simulink model "regulator"  (R2023a)
settings: Solver=VariableStepAuto  StartTime=0.0  StopTime=1250  RelTol=1e-3
values from neighbouring files (symbols this model uses):
  A = [   a11,    0,      0,      0 ... (first row only)    [linearize_4tanks.m]    (also in parameters.mat = [-0.0171366511824 0.0171366511824 0 0 0 -0.0952465397017 0 0)
  A_kf = [-0.0171366511824 0.0171366511824 0 0 -0.405989384527 -1.0114279511 -4.63493813994e-17 -1.85727570483e-16 0 0 -0.052376732387 0.052376732387 ... (16 elements, 4x4)]    [parameters.mat]
  B = [   0,      b12 ... (first row only)    [linearize_4tanks.m]    (also in parameters.mat = [0  0.0970102697521; 0.120715699163  0; 0.138722651778  0; 0)
  B_kf = [0 0.120715699163 0.138722651778 0 0.0970102697521 0 0 0.159450121706 0.405989384527 0.916181411394 4.63493813994e-17 1.85727570483e-16 ... (16 elements, 4x4)]    [parameters.mat]
  C = [   0,      1,      0,      0 ... (first row only)    [linearize_4tanks.m]    (also in parameters.mat = [0  1  0  0; 0  0  0  1])
  C_kf = [1 0 0 0 0 1 0 0 0 0 1 0 ... (16 elements, 4x4)]    [parameters.mat]
  D_kf = [0 0 0 0 0 0 0 0 0 0 0 0 ... (16 elements, 4x4)]    [parameters.mat]
  K_integrators = [-0.0995479981451  -0.00949716090787; 0.00949716090787  -0.0995479981451]    [parameters.mat]
  K_state = [0.12950650673  0.722856465098  0.0139705767535  0.0637209208421; -0.0211766819284  -0.0833619871599  0.236348353203  0.657206774714]    [parameters.mat]
  u_bar = reshape(z_opt(5:6), [2, 1])    [linearize_4tanks.m]    (also in parameters.mat = [6.60003195923 9.28189672086])
  x_bar = reshape(z_opt(1:4), [4, 1])    [linearize_4tanks.m]    (also in parameters.mat = [24.6597369405 10 3.03378366821 10])
undefined symbols (not defined in the file or in its folder): DiscIntNeverNeededParam
libraries: discretizing x2
settings Model: Creator=ermarinellone  LastModifiedBy=ermarinellone

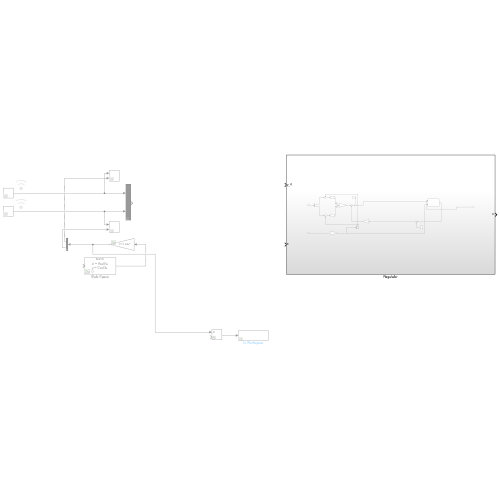
[thumbnail: Simulink's stored preview of the top-level diagram]
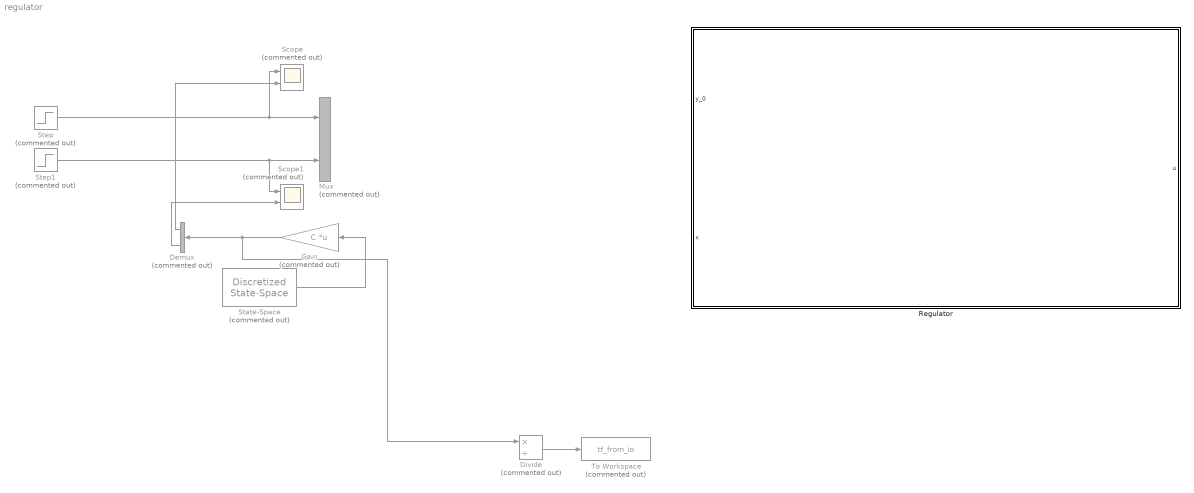
== system regulator ==
  Demux : Demux  Commented=on  Outputs=2
  Divide : Product  Commented=on  Inputs=*/
  Gain : Gain  Commented=on  Gain=C  Multiplication=Matrix(K*u) (u vector)
  Mux : Mux  Commented=on  Inputs=2
  Regulator : Subsystem
  Scope : Scope  Commented=on  NumInputPorts=2
  Scope1 : Scope  Commented=on  NumInputPorts=2
  State-Space : discretizing/Discretized State-Space  Commented=on  A=A  B=B  C=eye(4)  D=zeros(4,2)  ic=0  AbsTol=auto  SampleTime=0.01  method=tustin  Wc=1
  Step : Step  Commented=on  Time=500  Before=10  After=13  SampleTime=0
  Step1 : Step  Commented=on  Time=500  Before=10  After=10  SampleTime=0
  To Workspace : ToWorkspace  Commented=on  VariableName=tf_from_io  SaveFormat=Timeseries  SampleTime=-1
  wires:
  State-Space/1 -> Gain/1
  Demux/1 -> Scope/2
  Demux/2 -> Scope1/2
  Gain/1 -> Divide/1, Demux/1
  Step/1 -> Scope/1, Mux/1
  Step1/1 -> Scope1/1, Mux/2
  Divide/1 -> To Workspace/1

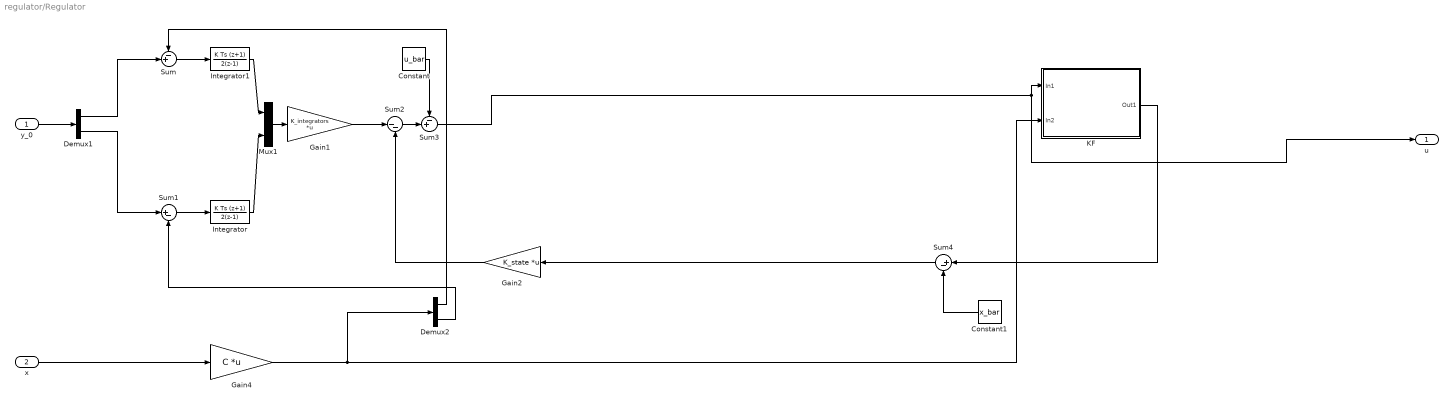
== system regulator/Regulator ==
  y_0 : Inport
  x : Inport  Port=2
  Constant : Constant  Value=u_bar
  Constant1 : Constant  Value=x_bar
  Demux1 : Demux  Outputs=2
  Demux2 : Demux  Outputs=2
  Gain1 : Gain  Gain=K_integrators  Multiplication=Matrix(K*u) (u vector)
  Gain2 : Gain  Gain=K_state  Multiplication=Matrix(K*u) (u vector)
  Gain4 : Gain  Gain=C  Multiplication=Matrix(K*u) (u vector)
  Integrator : DiscreteIntegrator  IntegratorMethod=Integration: Trapezoidal  SampleTime=0.01  ICPrevOutput=DiscIntNeverNeededParam  ICPrevScaledInput=DiscIntNeverNeededParam  mask(DiscretizedDiscreteIntegrator){}
      mask init:
      | %tustin
  Integrator1 : DiscreteIntegrator  IntegratorMethod=Integration: Trapezoidal  SampleTime=0.01  ICPrevOutput=DiscIntNeverNeededParam  ICPrevScaledInput=DiscIntNeverNeededParam  mask(DiscretizedDiscreteIntegrator){}
      mask init:
      | %tustin
  KF : Subsystem
  Mux1 : Mux  Inputs=2
  Sum : Sum  Inputs=-+|
  Sum1 : Sum  Inputs=|+-
  Sum2 : Sum  Inputs=|--
  Sum3 : Sum  Inputs=-+|
  Sum4 : Sum  Inputs=|+-
  u : Outport
  wires:
  Sum4/1 -> Gain2/1
  Sum/1 -> Integrator1/1
  KF/1(Out1) -> Sum4/1
  Sum1/1 -> Integrator/1
  Gain4/1 -> Demux2/1, KF/2(In2)
  Constant1/1 -> Sum4/2
  Sum2/1 -> Sum3/2
  Gain1/1 -> Sum2/1
  Integrator/1 -> Mux1/2
  Mux1/1 -> Gain1/1
  Constant/1 -> Sum3/1
  Sum3/1 -> KF/1(In1), u/1
  Gain2/1 -> Sum2/2
  Integrator1/1 -> Mux1/1
  x/1 -> Gain4/1
  y_0/1 -> Demux1/1
  Demux1/1 -> Sum/2
  Demux1/2 -> Sum1/1
  Demux2/1 -> Sum/1
  Demux2/2 -> Sum1/2

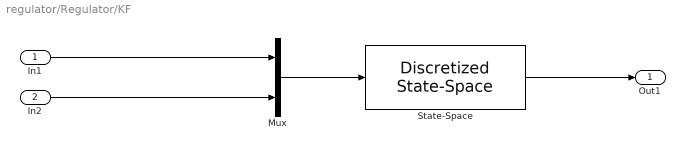
== system regulator/Regulator/KF ==
  In1 : Inport
  In2 : Inport  Port=2
  Mux : Mux  Inputs=2
  State-Space : discretizing/Discretized State-Space  A=A_kf  B=B_kf  C=C_kf  D=D_kf  ic=0  AbsTol=auto  SampleTime=0.01  method=tustin  Wc=1
  Out1 : Outport
  wires:
  In1/1 -> Mux/1
  Mux/1 -> State-Space/1
  State-Space/1 -> Out1/1
  In2/1 -> Mux/2
